simulink model "IEEE33BusTestSystemSimple"  (Simulink 10.3)
settings: Solver=FixedStepAuto  StartTime=0.0  StopTime=0.2  RelTol=1e-3
undefined symbols (not defined in the file): D1, Delta
libraries: spsThreePhaseVIMeasurementLib x43, spsThreePhaseSeriesRLCBranchLib x39, spsThreePhaseSeriesRLCLoadLib x34, simulink_extras x9, spsFrequencyPhasorLib x9, spsPowerPositiveSequenceLib x9, spsSequenceAnalyzerLib x9, spsThreePhaseParallelRLCLoadLib x3, spsSeriesRLCBranchLib x3, spsAC1AExcitationSystemLib x2, spsDieselMotorModel x2, spsSynchronousMachinepuStandardLib x2
(part 3 of 3)

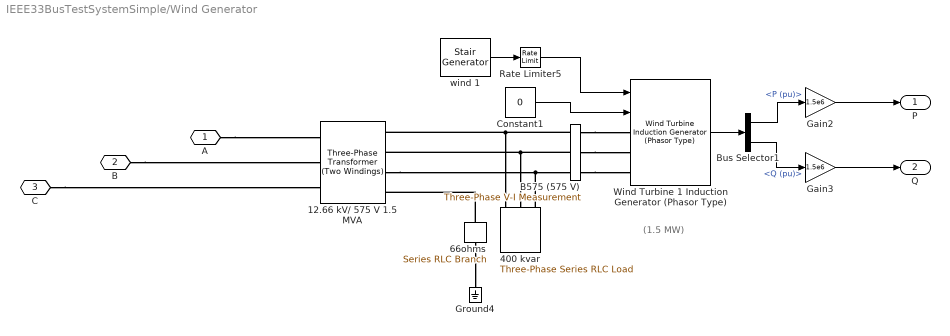
== system IEEE33BusTestSystemSimple/Wind Generator ==
  note: (1.5 MW)
  12.66 kV/ 575 V 1.5 MVA : spsThreePhaseTransformerTwoWindingsLib/Three-Phase Transformer (Two Windings)  Winding1Connection=Yg  Winding2Connection=Yn  CoreType=Three single-phase transformers  SetSaturation=off  Hysteresis=off  DataFile='hysteresis'  SetInitialFlux=off  Measurements=None  UNITS=pu  NominalPower="[1.5e6  50]"  Winding1=[12.66e3 , 0.025/30 , 0.025]  Winding2=[ 575, 0.025/30 , 0.025]  Rm=500  Lm=inf  L0=0.5  Saturation=[ 0,0 ; 0.0024,1.2 ; 1.0,1.52 ]  InitialFluxes=[ 0.8 , -0.8 , 0.7 ]  BreakLoop=off  DiscreteSolver=Trapezoidal iterative  DataType=off  TransfoNumber=0
  400 kvar : spsThreePhaseSeriesRLCLoadLib/Three-Phase Series RLC Load  LConnTagsString=A|B|C  Configuration=Delta  NominalVoltage=575  Vabc=[1e3 1e3 1e3]  Vabcp=[1e3 1e3 1e3]  NominalFrequency=50  UnbalancedPower=off  ActivePower=0  InductivePower=0  CapacitivePower=400e3  Pabc=[10e3 9e3 11e3]  QLabc=[100 90 110]  QCabc=[100 90 110]  Pabcp=[10e3 9e3 11e3]  QLabcp=[100 90 110]  QCabcp=[100 90 110]  Measurements=None  LoadType=constant Z
  "66ohms " : spsSeriesRLCBranchLib/Series RLC Branch  LConnTagsString=__new0  RConnTagsString=__new0  BranchType=R  Resistance=66  Inductance=1.0  SetiL0=off  InitialCurrent=0  Capacitance=1.0  Setx0=off  InitialVoltage=0  Measurements=None
  B575 (575 V) : spsThreePhaseVIMeasurementLib/Three-Phase V-I Measurement  VoltageMeasurement=phase-to-ground  SetLabelV=on  LabelV=Vabc_B575  Vpu=on  VpuLL=off  CurrentMeasurement=yes  SetLabelI=on  LabelI=Iabc_B575  Ipu=on  Pbase=1.5e6/0.9  Vbase=575  OutputType=Complex  PhasorSimulation=off  PSBequivalent=0
  Bus Selector1 : BusSelector  OutputSignals=P (pu),Q (pu)
  Constant1 : Constant  Value=0
  Gain2 : Gain  Gain=1.5e6
  Gain3 : Gain  Gain=1.5e6
  Ground4 : spsGroundLib/Ground  LConnTagsString=a
  Rate Limiter5 : RateLimiter
  Wind Turbine 1 Induction Generator (Phasor Type) : spsWindTurbineInductionGeneratorPhasorTypeLib/Wind Turbine Induction Generator (Phasor Type)  ExternalTm=off  nom=[1.5e6/0.9 575 50]  sta=[ 0.004843 0.1248]  rot=[ 0.004377 0.1791]  Lm=6.77  mec=[5.04 0.01 3]  init="[ -0.01,0   0,0,0   0,0,0 ]"  pitch_angle=0  Pmec=1.5e6  wind_base=9  speed_nom=1  P_wind_base=1  K_pitch_gain=[5 25]  pitch_max=45  pitch_rate=2
      settings: SourceProductBaseCode=PS
  wind 1 : spsStairGeneratorLib/Stair Generator  t=[ 0 2]  e=[8 12]  Ts=0
  A : PMIOPort  Side=Left
  B : PMIOPort  Port=2  Side=Left
  C : PMIOPort  Port=3  Side=Left
  P : Outport  VectorParamsAs1DForOutWhenUnconnected=off
  Q : Outport  Port=2  VectorParamsAs1DForOutWhenUnconnected=off
  wires:
  wind 1/1 -> Rate Limiter5/1
  Constant1/1 -> Wind Turbine 1 Induction Generator (Phasor Type)/2
  Rate Limiter5/1 -> Wind Turbine 1 Induction Generator (Phasor Type)/1
  Wind Turbine 1 Induction Generator (Phasor Type)/1 -> Bus Selector1/1
  Bus Selector1/1 -> Gain2/1  "<P (pu)>"
  Gain2/1 -> P/1
  Bus Selector1/2 -> Gain3/1  "<Q (pu)>"
  Gain3/1 -> Q/1
  connections:
  A/RConn1 -- 12.66 kV/ 575 V 1.5 MVA/LConn1
  12.66 kV/ 575 V 1.5 MVA/RConn3 -- 400 kvar/LConn3 -- B575 (575 V)/LConn3
  "66ohms "/RConn1 -- Ground4/LConn1
  B575 (575 V)/LConn2 -- 400 kvar/LConn2 -- 12.66 kV/ 575 V 1.5 MVA/RConn2
  B575 (575 V)/LConn1 -- 400 kvar/LConn1 -- 12.66 kV/ 575 V 1.5 MVA/RConn1
  "66ohms "/LConn1 -- 12.66 kV/ 575 V 1.5 MVA/RConn4
  B575 (575 V)/RConn3 -- Wind Turbine 1 Induction Generator (Phasor Type)/LConn3
  B575 (575 V)/RConn1 -- Wind Turbine 1 Induction Generator (Phasor Type)/LConn1
  B575 (575 V)/RConn2 -- Wind Turbine 1 Induction Generator (Phasor Type)/LConn2
  C/RConn1 -- 12.66 kV/ 575 V 1.5 MVA/LConn3
  B/RConn1 -- 12.66 kV/ 575 V 1.5 MVA/LConn2

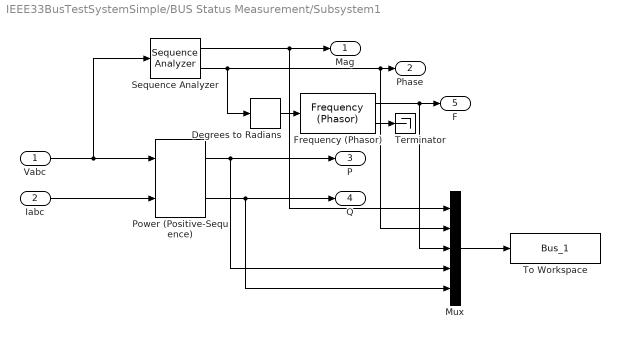
== system IEEE33BusTestSystemSimple/BUS Status Measurement/Subsystem1 ==
  Vabc : Inport
  Iabc : Inport  Port=2
  Degrees to Radians : simulink_extras/Transformations/Degrees to Radians
  Frequency (Phasor) : spsFrequencyPhasorLib/Frequency (Phasor)  Fn=50  T=0.1
      settings: SourceProductBaseCode=PS
  Mux : Mux  Inputs=5
  Power (Positive-Sequence) : spsPowerPositiveSequenceLib/Power (Positive-Sequence)  Freq=50  Vinit=[0, 0]  Iinit=[0, 0]  Ts=0
      settings: SourceProductBaseCode=PS
  Sequence Analyzer : spsSequenceAnalyzerLib/Sequence Analyzer  Freq=50  n=1  seq=Positive  InInit=[0, 0]  Ts=0
      settings: SourceProductBaseCode=PS
  Terminator : Terminator
  To Workspace : ToWorkspace  VariableName=Bus_1  SaveFormat=Timeseries  SampleTime=-1
  Mag : Outport
  Phase : Outport  Port=2
  P : Outport  Port=3
  Q : Outport  Port=4
  F : Outport  Port=5
  wires:
  Vabc/1 -> Sequence Analyzer/1, Power (Positive-Sequence)/1
  Power (Positive-Sequence)/2 -> Q/1, Mux/5
  Iabc/1 -> Power (Positive-Sequence)/2
  Power (Positive-Sequence)/1 -> P/1, Mux/4
  Sequence Analyzer/2 -> Mux/2, Phase/1, Degrees to Radians/1
  Sequence Analyzer/1 -> Mux/1, Mag/1
  Degrees to Radians/1 -> Frequency (Phasor)/1
  Frequency (Phasor)/1 -> Mux/3, F/1
  Frequency (Phasor)/2 -> Terminator/1
  Mux/1 -> To Workspace/1

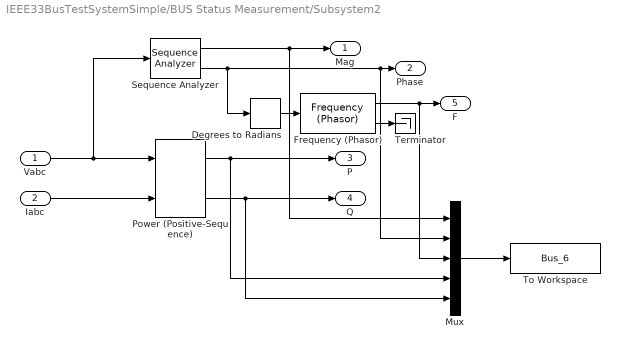
== system IEEE33BusTestSystemSimple/BUS Status Measurement/Subsystem2 ==
  Vabc : Inport
  Iabc : Inport  Port=2
  Degrees to Radians : simulink_extras/Transformations/Degrees to Radians
  Frequency (Phasor) : spsFrequencyPhasorLib/Frequency (Phasor)  Fn=50  T=0.1
      settings: SourceProductBaseCode=PS
  Mux : Mux  Inputs=5
  Power (Positive-Sequence) : spsPowerPositiveSequenceLib/Power (Positive-Sequence)  Freq=50  Vinit=[0, 0]  Iinit=[0, 0]  Ts=0
      settings: SourceProductBaseCode=PS
  Sequence Analyzer : spsSequenceAnalyzerLib/Sequence Analyzer  Freq=50  n=1  seq=Positive  InInit=[0, 0]  Ts=0
      settings: SourceProductBaseCode=PS
  Terminator : Terminator
  To Workspace : ToWorkspace  VariableName=Bus_6  SaveFormat=Timeseries  SampleTime=-1
  Mag : Outport
  Phase : Outport  Port=2
  P : Outport  Port=3
  Q : Outport  Port=4
  F : Outport  Port=5
  wires:
  Vabc/1 -> Sequence Analyzer/1, Power (Positive-Sequence)/1
  Iabc/1 -> Power (Positive-Sequence)/2
  Degrees to Radians/1 -> Frequency (Phasor)/1
  Frequency (Phasor)/2 -> Terminator/1
  Sequence Analyzer/1 -> Mux/1, Mag/1
  Mux/1 -> To Workspace/1
  Power (Positive-Sequence)/2 -> Mux/5, Q/1
  Frequency (Phasor)/1 -> Mux/3, F/1
  Sequence Analyzer/2 -> Mux/2, Phase/1, Degrees to Radians/1
  Power (Positive-Sequence)/1 -> Mux/4, P/1

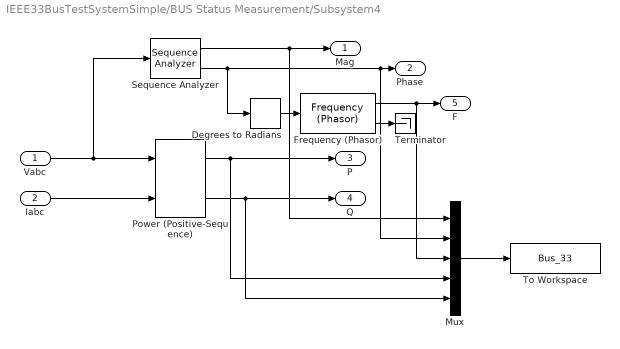
== system IEEE33BusTestSystemSimple/BUS Status Measurement/Subsystem4 ==
  Vabc : Inport
  Iabc : Inport  Port=2
  Degrees to Radians : simulink_extras/Transformations/Degrees to Radians
  Frequency (Phasor) : spsFrequencyPhasorLib/Frequency (Phasor)  Fn=50  T=0.1
      settings: SourceProductBaseCode=PS
  Mux : Mux  Inputs=5
  Power (Positive-Sequence) : spsPowerPositiveSequenceLib/Power (Positive-Sequence)  Freq=50  Vinit=[0, 0]  Iinit=[0, 0]  Ts=0
      settings: SourceProductBaseCode=PS
  Sequence Analyzer : spsSequenceAnalyzerLib/Sequence Analyzer  Freq=50  n=1  seq=Positive  InInit=[0, 0]  Ts=0
      settings: SourceProductBaseCode=PS
  Terminator : Terminator
  To Workspace : ToWorkspace  VariableName=Bus_33  SaveFormat=Timeseries  SampleTime=-1
  Mag : Outport
  Phase : Outport  Port=2
  P : Outport  Port=3
  Q : Outport  Port=4
  F : Outport  Port=5
  wires:
  Vabc/1 -> Sequence Analyzer/1, Power (Positive-Sequence)/1
  Iabc/1 -> Power (Positive-Sequence)/2
  Degrees to Radians/1 -> Frequency (Phasor)/1
  Frequency (Phasor)/2 -> Terminator/1
  Sequence Analyzer/1 -> Mux/1, Mag/1
  Mux/1 -> To Workspace/1
  Power (Positive-Sequence)/2 -> Mux/5, Q/1
  Frequency (Phasor)/1 -> Mux/3, F/1
  Sequence Analyzer/2 -> Mux/2, Phase/1, Degrees to Radians/1
  Power (Positive-Sequence)/1 -> Mux/4, P/1

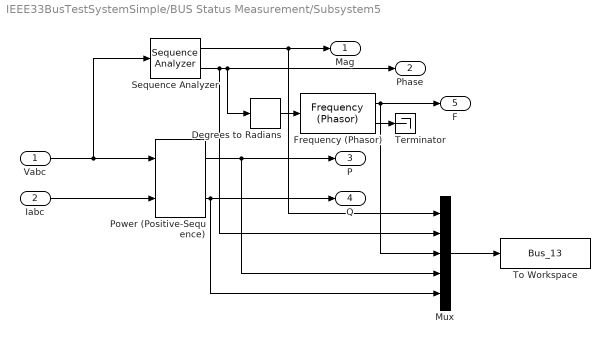
== system IEEE33BusTestSystemSimple/BUS Status Measurement/Subsystem5 ==
  Vabc : Inport
  Iabc : Inport  Port=2
  Degrees to Radians : simulink_extras/Transformations/Degrees to Radians
  Frequency (Phasor) : spsFrequencyPhasorLib/Frequency (Phasor)  Fn=50  T=0.1
      settings: SourceProductBaseCode=PS
  Mux : Mux  Inputs=5
  Power (Positive-Sequence) : spsPowerPositiveSequenceLib/Power (Positive-Sequence)  Freq=50  Vinit=[0, 0]  Iinit=[0, 0]  Ts=0
      settings: SourceProductBaseCode=PS
  Sequence Analyzer : spsSequenceAnalyzerLib/Sequence Analyzer  Freq=50  n=1  seq=Positive  InInit=[0, 0]  Ts=0
      settings: SourceProductBaseCode=PS
  Terminator : Terminator
  To Workspace : ToWorkspace  VariableName=Bus_13  SaveFormat=Timeseries  SampleTime=-1
  Mag : Outport
  Phase : Outport  Port=2
  P : Outport  Port=3
  Q : Outport  Port=4
  F : Outport  Port=5
  wires:
  Vabc/1 -> Sequence Analyzer/1, Power (Positive-Sequence)/1
  Iabc/1 -> Power (Positive-Sequence)/2
  Degrees to Radians/1 -> Frequency (Phasor)/1
  Frequency (Phasor)/2 -> Terminator/1
  Sequence Analyzer/1 -> Mux/1, Mag/1
  Mux/1 -> To Workspace/1
  Power (Positive-Sequence)/2 -> Mux/5, Q/1
  Frequency (Phasor)/1 -> Mux/3, F/1
  Sequence Analyzer/2 -> Mux/2, Phase/1, Degrees to Radians/1
  Power (Positive-Sequence)/1 -> Mux/4, P/1

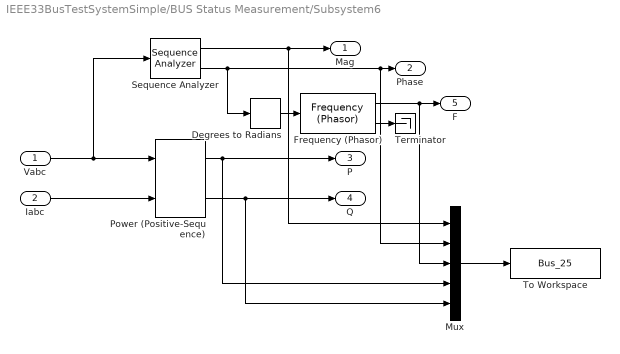
== system IEEE33BusTestSystemSimple/BUS Status Measurement/Subsystem6 ==
  Vabc : Inport
  Iabc : Inport  Port=2
  Degrees to Radians : simulink_extras/Transformations/Degrees to Radians
  Frequency (Phasor) : spsFrequencyPhasorLib/Frequency (Phasor)  Fn=50  T=0.1
      settings: SourceProductBaseCode=PS
  Mux : Mux  Inputs=5
  Power (Positive-Sequence) : spsPowerPositiveSequenceLib/Power (Positive-Sequence)  Freq=50  Vinit=[0, 0]  Iinit=[0, 0]  Ts=0
      settings: SourceProductBaseCode=PS
  Sequence Analyzer : spsSequenceAnalyzerLib/Sequence Analyzer  Freq=50  n=1  seq=Positive  InInit=[0, 0]  Ts=0
      settings: SourceProductBaseCode=PS
  Terminator : Terminator
  To Workspace : ToWorkspace  VariableName=Bus_25  SaveFormat=Timeseries  SampleTime=-1
  Mag : Outport
  Phase : Outport  Port=2
  P : Outport  Port=3
  Q : Outport  Port=4
  F : Outport  Port=5
  wires:
  Vabc/1 -> Sequence Analyzer/1, Power (Positive-Sequence)/1
  Iabc/1 -> Power (Positive-Sequence)/2
  Degrees to Radians/1 -> Frequency (Phasor)/1
  Frequency (Phasor)/2 -> Terminator/1
  Sequence Analyzer/1 -> Mux/1, Mag/1
  Mux/1 -> To Workspace/1
  Power (Positive-Sequence)/2 -> Mux/5, Q/1
  Frequency (Phasor)/1 -> Mux/3, F/1
  Sequence Analyzer/2 -> Mux/2, Phase/1, Degrees to Radians/1
  Power (Positive-Sequence)/1 -> Mux/4, P/1

== system IEEE33BusTestSystemSimple/Bus_10/VI Recorder13 ==
  Vrec : Inport
  Irec : Inport  Port=2
  tag scope: I9to10=global, V9to10=global
  wires:
  Vrec/1 -> [V9to10]
  Irec/1 -> [I9to10]

== system IEEE33BusTestSystemSimple/Bus_11/VI Recorder14 ==
  Vrec : Inport
  Irec : Inport  Port=2
  tag scope: I10to11=global, V10to11=global
  wires:
  Vrec/1 -> [V10to11]
  Irec/1 -> [I10to11]

== system IEEE33BusTestSystemSimple/Bus_12/VI Recorder15 ==
  Vrec : Inport
  Irec : Inport  Port=2
  tag scope: I11to12=global, V11to12=global
  wires:
  Vrec/1 -> [V11to12]
  Irec/1 -> [I11to12]

== system IEEE33BusTestSystemSimple/Bus_13/VI Recorder16 ==
  Vrec : Inport
  Irec : Inport  Port=2
  tag scope: I12to13=global, V12to13=global
  wires:
  Vrec/1 -> [V12to13]
  Irec/1 -> [I12to13]

== system IEEE33BusTestSystemSimple/Bus_14/VI Recorder17 ==
  Vrec : Inport
  Irec : Inport  Port=2
  tag scope: I13to14=global, V13to14=global
  wires:
  Vrec/1 -> [V13to14]
  Irec/1 -> [I13to14]

== system IEEE33BusTestSystemSimple/Bus_15/VI Recorder18 ==
  Vrec : Inport
  Irec : Inport  Port=2
  tag scope: I14to15=global, V14to15=global
  wires:
  Vrec/1 -> [V14to15]
  Irec/1 -> [I14to15]

== system IEEE33BusTestSystemSimple/Bus_16/VI Recorder19 ==
  Vrec : Inport
  Irec : Inport  Port=2
  tag scope: I15to16=global, V15to16=global
  wires:
  Vrec/1 -> [V15to16]
  Irec/1 -> [I15to16]

== system IEEE33BusTestSystemSimple/Bus_17/VI Recorder20 ==
  Vrec : Inport
  Irec : Inport  Port=2
  tag scope: I16to17=global, V16to17=global
  wires:
  Vrec/1 -> [V16to17]
  Irec/1 -> [I16to17]

== system IEEE33BusTestSystemSimple/Bus_18/VI Recorder21 ==
  Vrec : Inport
  Irec : Inport  Port=2
  tag scope: I17to18=global, V17to18=global
  wires:
  Vrec/1 -> [V17to18]
  Irec/1 -> [I17to18]

== system IEEE33BusTestSystemSimple/Bus_19/VI Recorder ==
  Vrec : Inport
  Irec : Inport  Port=2
  tag scope: I2to19=global, V2to19=global
  wires:
  Vrec/1 -> [V2to19]
  Irec/1 -> [I2to19]

== system IEEE33BusTestSystemSimple/Bus_2/VI Recorder5 ==
  Vrec : Inport
  Irec : Inport  Port=2
  tag scope: I1to2=global, V1to2=global
  wires:
  Vrec/1 -> [V1to2]
  Irec/1 -> [I1to2]

== system IEEE33BusTestSystemSimple/Bus_20/VI Recorder1 ==
  Vrec : Inport
  Irec : Inport  Port=2
  tag scope: I19to20=global, V19to20=global
  wires:
  Vrec/1 -> [V19to20]
  Irec/1 -> [I19to20]

== system IEEE33BusTestSystemSimple/Bus_21/VI Recorder2 ==
  Vrec : Inport
  Irec : Inport  Port=2
  tag scope: I20to21=global, V20to21=global
  wires:
  Vrec/1 -> [V20to21]
  Irec/1 -> [I20to21]

== system IEEE33BusTestSystemSimple/Bus_22/VI Recorder3 ==
  Vrec : Inport
  Irec : Inport  Port=2
  tag scope: I21to22=global, V21to22=global
  wires:
  Vrec/1 -> [V21to22]
  Irec/1 -> [I21to22]

== system IEEE33BusTestSystemSimple/Bus_23/VI Recorder32 ==
  Vrec : Inport
  Irec : Inport  Port=2
  tag scope: I3to23=global, V3to23=global
  wires:
  Vrec/1 -> [V3to23]
  Irec/1 -> [I3to23]

== system IEEE33BusTestSystemSimple/Bus_24/VI Recorder31 ==
  Vrec : Inport
  Irec : Inport  Port=2
  tag scope: I23to24=global, V23to24=global
  wires:
  Vrec/1 -> [V23to24]
  Irec/1 -> [I23to24]

== system IEEE33BusTestSystemSimple/Bus_25/VI Recorder30 ==
  Vrec : Inport
  Irec : Inport  Port=2
  tag scope: I24to25=global, V24to25=global
  wires:
  Vrec/1 -> [V24to25]
  Irec/1 -> [I24to25]

== system IEEE33BusTestSystemSimple/Bus_26/VI Recorder22 ==
  Vrec : Inport
  Irec : Inport  Port=2
  tag scope: I6to26=global, V6to26=global
  wires:
  Vrec/1 -> [V6to26]
  Irec/1 -> [I6to26]

== system IEEE33BusTestSystemSimple/Bus_27/VI Recorder23 ==
  Vrec : Inport
  Irec : Inport  Port=2
  tag scope: I26to27=global, V26to27=global
  wires:
  Vrec/1 -> [V26to27]
  Irec/1 -> [I26to27]

== system IEEE33BusTestSystemSimple/Bus_28/VI Recorder24 ==
  Vrec : Inport
  Irec : Inport  Port=2
  tag scope: I27to28=global, V27to28=global
  wires:
  Vrec/1 -> [V27to28]
  Irec/1 -> [I27to28]

== system IEEE33BusTestSystemSimple/Bus_29/VI Recorder25 ==
  Vrec : Inport
  Irec : Inport  Port=2
  tag scope: I28to29=global, V28to29=global
  wires:
  Vrec/1 -> [V28to29]
  Irec/1 -> [I28to29]

== system IEEE33BusTestSystemSimple/Bus_3/VI Recorder6 ==
  Vrec : Inport
  Irec : Inport  Port=2
  tag scope: I2to3=global, V2to3=global
  wires:
  Vrec/1 -> [V2to3]
  Irec/1 -> [I2to3]

== system IEEE33BusTestSystemSimple/Bus_30/VI Recorder26 ==
  Vrec : Inport
  Irec : Inport  Port=2
  tag scope: I29to30=global, V29to30=global
  wires:
  Vrec/1 -> [V29to30]
  Irec/1 -> [I29to30]

== system IEEE33BusTestSystemSimple/Bus_31/VI Recorder27 ==
  Vrec : Inport
  Irec : Inport  Port=2
  tag scope: I30to31=global, V30to31=global
  wires:
  Vrec/1 -> [V30to31]
  Irec/1 -> [I30to31]

== system IEEE33BusTestSystemSimple/Bus_32/VI Recorder28 ==
  Vrec : Inport
  Irec : Inport  Port=2
  tag scope: I31to32=global, V31to32=global
  wires:
  Vrec/1 -> [V31to32]
  Irec/1 -> [I31to32]

== system IEEE33BusTestSystemSimple/Bus_33/VI Recorder29 ==
  Vrec : Inport
  Irec : Inport  Port=2
  tag scope: I32to33=global, V32to33=global
  wires:
  Vrec/1 -> [V32to33]
  Irec/1 -> [I32to33]

== system IEEE33BusTestSystemSimple/Bus_4/VI Recorder7 ==
  Vrec : Inport
  Irec : Inport  Port=2
  tag scope: I3to4=global, V3to4=global
  wires:
  Vrec/1 -> [V3to4]
  Irec/1 -> [I3to4]

== system IEEE33BusTestSystemSimple/Bus_5/VI Recorder8 ==
  Vrec : Inport
  Irec : Inport  Port=2
  tag scope: I4to5=global, V4to5=global
  wires:
  Vrec/1 -> [V4to5]
  Irec/1 -> [I4to5]

== system IEEE33BusTestSystemSimple/Bus_6/VI Recorder9 ==
  Vrec : Inport
  Irec : Inport  Port=2
  tag scope: I5to6=global, V5to6=global
  wires:
  Vrec/1 -> [V5to6]
  Irec/1 -> [I5to6]

== system IEEE33BusTestSystemSimple/Bus_7/VI Recorder10 ==
  Vrec : Inport
  Irec : Inport  Port=2
  tag scope: I6to7=global, V6to7=global
  wires:
  Vrec/1 -> [V6to7]
  Irec/1 -> [I6to7]

== system IEEE33BusTestSystemSimple/Bus_8/VI Recorder11 ==
  Vrec : Inport
  Irec : Inport  Port=2
  tag scope: I7to8=global, V7to8=global
  wires:
  Vrec/1 -> [V7to8]
  Irec/1 -> [I7to8]

== system IEEE33BusTestSystemSimple/Bus_9/VI Recorder12 ==
  Vrec : Inport
  Irec : Inport  Port=2
  tag scope: I8to9=global, V8to9=global
  wires:
  Vrec/1 -> [V8to9]
  Irec/1 -> [I8to9]

== system IEEE33BusTestSystemSimple/DG Systems Status/Subsystem1 ==
  Vabc : Inport
  Iabc : Inport  Port=2
  Degrees to Radians : simulink_extras/Transformations/Degrees to Radians
  Frequency (Phasor) : spsFrequencyPhasorLib/Frequency (Phasor)  Fn=50  T=0.1
      settings: SourceProductBaseCode=PS
  Power (Positive-Sequence) : spsPowerPositiveSequenceLib/Power (Positive-Sequence)  Freq=50  Vinit=[0, 0]  Iinit=[0, 0]  Ts=0
      settings: SourceProductBaseCode=PS
  Sequence Analyzer : spsSequenceAnalyzerLib/Sequence Analyzer  Freq=50  n=1  seq=Positive  InInit=[0, 0]  Ts=0
      settings: SourceProductBaseCode=PS
  Terminator : Terminator
  Mag : Outport
  Phase : Outport  Port=2
  P : Outport  Port=3
  Q : Outport  Port=4
  F : Outport  Port=5
  wires:
  Vabc/1 -> Sequence Analyzer/1, Power (Positive-Sequence)/1
  Power (Positive-Sequence)/2 -> Q/1
  Iabc/1 -> Power (Positive-Sequence)/2
  Power (Positive-Sequence)/1 -> P/1
  Sequence Analyzer/2 -> Phase/1, Degrees to Radians/1
  Sequence Analyzer/1 -> Mag/1
  Degrees to Radians/1 -> Frequency (Phasor)/1
  Frequency (Phasor)/1 -> F/1
  Frequency (Phasor)/2 -> Terminator/1

== system IEEE33BusTestSystemSimple/DG Systems Status/Subsystem2 ==
  Vabc : Inport
  Iabc : Inport  Port=2
  Degrees to Radians : simulink_extras/Transformations/Degrees to Radians
  Frequency (Phasor) : spsFrequencyPhasorLib/Frequency (Phasor)  Fn=50  T=0.1
      settings: SourceProductBaseCode=PS
  Power (Positive-Sequence) : spsPowerPositiveSequenceLib/Power (Positive-Sequence)  Freq=50  Vinit=[0, 0]  Iinit=[0, 0]  Ts=0
      settings: SourceProductBaseCode=PS
  Sequence Analyzer : spsSequenceAnalyzerLib/Sequence Analyzer  Freq=50  n=1  seq=Positive  InInit=[0, 0]  Ts=0
      settings: SourceProductBaseCode=PS
  Terminator : Terminator
  Mag : Outport
  Phase : Outport  Port=2
  P : Outport  Port=3
  Q : Outport  Port=4
  F : Outport  Port=5
  wires:
  Vabc/1 -> Sequence Analyzer/1, Power (Positive-Sequence)/1
  Power (Positive-Sequence)/2 -> Q/1
  Iabc/1 -> Power (Positive-Sequence)/2
  Power (Positive-Sequence)/1 -> P/1
  Sequence Analyzer/2 -> Phase/1, Degrees to Radians/1
  Sequence Analyzer/1 -> Mag/1
  Degrees to Radians/1 -> Frequency (Phasor)/1
  Frequency (Phasor)/1 -> F/1
  Frequency (Phasor)/2 -> Terminator/1

== system IEEE33BusTestSystemSimple/DG Systems Status/Subsystem3 ==
  Vabc : Inport
  Iabc : Inport  Port=2
  Degrees to Radians : simulink_extras/Transformations/Degrees to Radians
  Frequency (Phasor) : spsFrequencyPhasorLib/Frequency (Phasor)  Fn=50  T=0.1
      settings: SourceProductBaseCode=PS
  Power (Positive-Sequence) : spsPowerPositiveSequenceLib/Power (Positive-Sequence)  Freq=50  Vinit=[0, 0]  Iinit=[0, 0]  Ts=0
      settings: SourceProductBaseCode=PS
  Sequence Analyzer : spsSequenceAnalyzerLib/Sequence Analyzer  Freq=50  n=1  seq=Positive  InInit=[0, 0]  Ts=0
      settings: SourceProductBaseCode=PS
  Terminator : Terminator
  Mag : Outport
  Phase : Outport  Port=2
  P : Outport  Port=3
  Q : Outport  Port=4
  F : Outport  Port=5
  wires:
  Vabc/1 -> Sequence Analyzer/1, Power (Positive-Sequence)/1
  Power (Positive-Sequence)/2 -> Q/1
  Iabc/1 -> Power (Positive-Sequence)/2
  Power (Positive-Sequence)/1 -> P/1
  Sequence Analyzer/2 -> Phase/1, Degrees to Radians/1
  Sequence Analyzer/1 -> Mag/1
  Degrees to Radians/1 -> Frequency (Phasor)/1
  Frequency (Phasor)/1 -> F/1
  Frequency (Phasor)/2 -> Terminator/1

== system IEEE33BusTestSystemSimple/DG Systems Status/Subsystem4 ==
  Vabc : Inport
  Iabc : Inport  Port=2
  Degrees to Radians : simulink_extras/Transformations/Degrees to Radians
  Frequency (Phasor) : spsFrequencyPhasorLib/Frequency (Phasor)  Fn=50  T=0.1
      settings: SourceProductBaseCode=PS
  Power (Positive-Sequence) : spsPowerPositiveSequenceLib/Power (Positive-Sequence)  Freq=50  Vinit=[0, 0]  Iinit=[0, 0]  Ts=0
      settings: SourceProductBaseCode=PS
  Sequence Analyzer : spsSequenceAnalyzerLib/Sequence Analyzer  Freq=50  n=1  seq=Positive  InInit=[0, 0]  Ts=0
      settings: SourceProductBaseCode=PS
  Terminator : Terminator
  Mag : Outport
  Phase : Outport  Port=2
  P : Outport  Port=3
  Q : Outport  Port=4
  F : Outport  Port=5
  wires:
  Vabc/1 -> Sequence Analyzer/1, Power (Positive-Sequence)/1
  Power (Positive-Sequence)/2 -> Q/1
  Iabc/1 -> Power (Positive-Sequence)/2
  Power (Positive-Sequence)/1 -> P/1
  Sequence Analyzer/2 -> Phase/1, Degrees to Radians/1
  Sequence Analyzer/1 -> Mag/1
  Degrees to Radians/1 -> Frequency (Phasor)/1
  Frequency (Phasor)/1 -> F/1
  Frequency (Phasor)/2 -> Terminator/1

== system IEEE33BusTestSystemSimple/Diesel Generator 1/Generator Measures ==
  m : Inport
  Bus Selector : BusSelector  OutputSignals="dq0 components.Stator voltage  vq (pu),dq0 components.Stator voltage  vd (pu)"  OutputAsBus=on
  Bus Selector1 : BusSelector  OutputSignals="Mechanical.Rotor speed  wm  (pu),dq0 components.Field current  ifd (pu)"
  Fcn1 : Fcn  Expr=sqrt(u(1)^2 + u(2)^2)
  Ifd : Outport  VectorParamsAs1DForOutWhenUnconnected=off
  Vt : Outport  Port=2  VectorParamsAs1DForOutWhenUnconnected=off
  wm : Outport  Port=3  VectorParamsAs1DForOutWhenUnconnected=off
  wires:
  Bus Selector1/1 -> wm/1  "<Rotor speed  wm  (pu)>"
  m/1 -> Bus Selector1/1, Bus Selector/1
  Fcn1/1 -> Vt/1
  Bus Selector/1 -> Fcn1/1
  Bus Selector1/2 -> Ifd/1  "<Field current  ifd (pu)>"

== system IEEE33BusTestSystemSimple/Diesel Generator 1/Selected Measurements ==
  m : Inport
  Bus Creator : BusCreator  Inputs=7
  Bus Selector : BusSelector  OutputSignals="Mechanical.Electrical power  Pe (pu),Mechanical.Rotor speed  wm  (pu),Output active power   Peo (pu),Output reactive power  Qeo (pu)"
  to W : Gain  Gain=Pn
  to W1 : Gain  Gain=Pn
  to W2 : Gain  Gain=Pn
  sm : Outport  VectorParamsAs1DForOutWhenUnconnected=off
  wires:
  to W2/1 -> Bus Creator/7  "Reactive Power (W)"
  to W1/1 -> Bus Creator/6  "Active Power (W)"
  Bus Selector/2 -> Bus Creator/3  "<Rotor speed  wm  (pu)>"
  Bus Creator/1 -> sm/1
  to W/1 -> Bus Creator/1  "Electrical Power (W)"
  Bus Selector/3 -> Bus Creator/4, to W1/1  "<Output active power   Peo (pu)>"
  Bus Selector/1 -> to W/1, Bus Creator/2  "<Electrical power  Pe (pu)>"
  Bus Selector/4 -> Bus Creator/5, to W2/1  "<Output reactive power  Qeo (pu)>"
  m/1 -> Bus Selector/1

== system IEEE33BusTestSystemSimple/Diesel Generator 2/Generator Measures ==
  m : Inport
  Bus Selector : BusSelector  OutputSignals="dq0 components.Stator voltage  vq (pu),dq0 components.Stator voltage  vd (pu)"  OutputAsBus=on
  Bus Selector1 : BusSelector  OutputSignals="Mechanical.Rotor speed  wm  (pu),dq0 components.Field current  ifd (pu)"
  Fcn1 : Fcn  Expr=sqrt(u(1)^2 + u(2)^2)
  Ifd : Outport  VectorParamsAs1DForOutWhenUnconnected=off
  Vt : Outport  Port=2  VectorParamsAs1DForOutWhenUnconnected=off
  wm : Outport  Port=3  VectorParamsAs1DForOutWhenUnconnected=off
  wires:
  Bus Selector1/1 -> wm/1  "<Rotor speed  wm  (pu)>"
  m/1 -> Bus Selector1/1, Bus Selector/1
  Fcn1/1 -> Vt/1
  Bus Selector/1 -> Fcn1/1
  Bus Selector1/2 -> Ifd/1  "<Field current  ifd (pu)>"

== system IEEE33BusTestSystemSimple/Diesel Generator 2/Selected Measurements ==
  m : Inport
  Bus Creator : BusCreator  Inputs=7
  Bus Selector : BusSelector  OutputSignals="Mechanical.Electrical power  Pe (pu),Mechanical.Rotor speed  wm  (pu),Output active power   Peo (pu),Output reactive power  Qeo (pu)"
  to W : Gain  Gain=Pn
  to W1 : Gain  Gain=Pn
  to W2 : Gain  Gain=Pn
  sm : Outport  VectorParamsAs1DForOutWhenUnconnected=off
  wires:
  to W2/1 -> Bus Creator/7  "Reactive Power (W)"
  to W1/1 -> Bus Creator/6  "Active Power (W)"
  Bus Selector/2 -> Bus Creator/3  "<Rotor speed  wm  (pu)>"
  Bus Creator/1 -> sm/1
  to W/1 -> Bus Creator/1  "Electrical Power (W)"
  Bus Selector/3 -> Bus Creator/4, to W1/1  "<Output active power   Peo (pu)>"
  Bus Selector/1 -> to W/1, Bus Creator/2  "<Electrical power  Pe (pu)>"
  Bus Selector/4 -> Bus Creator/5, to W2/1  "<Output reactive power  Qeo (pu)>"
  m/1 -> Bus Selector/1

== system IEEE33BusTestSystemSimple/PV Array 2 /LC Filter ==
  C' : spsThreePhaseSeriesRLCBranchLib/Three-Phase Series RLC Branch  Commented=on  LConnTagsString=A|B|C  RConnTagsString=A|B|C  BranchType=C  Resistance=1e6  Inductance=500e-6/2  Capacitance=1e-3  Measurements=None
  L : spsThreePhaseSeriesRLCBranchLib/Three-Phase Series RLC Branch  LConnTagsString=A|B|C  RConnTagsString=A|B|C  BranchType=RL  Resistance=500e-6*377/50/2  Inductance=5*500e-6/2  Capacitance=inf  Measurements=None
  Three-Phase Series RLC Load : spsThreePhaseSeriesRLCLoadLib/Three-Phase Series RLC Load  LConnTagsString=A|B|C  Configuration=Y (grounded)  NominalVoltage=240  Vabc=[1e3 1e3 1e3]  Vabcp=[1e3 1e3 1e3]  NominalFrequency=50  UnbalancedPower=off  ActivePower=5*10e3/100  InductivePower=0  CapacitivePower=5*10e3  Pabc=[10e3 9e3 11e3]  QLabc=[100 90 110]  QCabc=[100 90 110]  Pabcp=[10e3 9e3 11e3]  QLabcp=[100 90 110]  QCabcp=[100 90 110]  Measurements=None  LoadType=constant Z
  A : PMIOPort  Side=Left
  a : PMIOPort  Port=2  Side=Right
  B : PMIOPort  Port=3  Side=Left
  b : PMIOPort  Port=4  Side=Right
  C : PMIOPort  Port=5  Side=Left
  c : PMIOPort  Port=6  Side=Right
  connections:
  c/RConn1 -- C'/LConn3 -- L/RConn3 -- Three-Phase Series RLC Load/LConn3
  C'/RConn1 -- C'/RConn3 -- C'/RConn2
  b/RConn1 -- L/RConn2 -- C'/LConn2 -- Three-Phase Series RLC Load/LConn2
  a/RConn1 -- C'/LConn1 -- L/RConn1 -- Three-Phase Series RLC Load/LConn1
  L/LConn3 -- C/RConn1
  L/LConn1 -- A/RConn1
  B/RConn1 -- L/LConn2

== system IEEE33BusTestSystemSimple/PV Array 2 /PWM ==
  Mux : Mux  Inputs=3
  PWM Generator (3-Level) : spsPWMGenerator3LevelLib/PWM Generator (3-Level)  ModulatorType=Three-phase bridge (12 pulses)  ModulatorMode=Unsynchronized  nF=27  Fc=27*50*3  ModulatingSignals=off  m=0.8  Freq=60  Phase=0  Ts=0
      settings: SourceProductBaseCode=PS
  Vref A : Sin  Frequency=2*pi*50  SampleTime=0
  Vref B : Sin  Frequency=2*pi*50  Phase=2*pi/3  SampleTime=0
  Vref C : Sin  Frequency=2*pi*50  Phase=4*pi/3  SampleTime=0
  pulse : Outport  VectorParamsAs1DForOutWhenUnconnected=off
  wires:
  Vref B/1 -> Mux/2
  Vref C/1 -> Mux/3
  PWM Generator (3-Level)/1 -> pulse/1
  Vref A/1 -> Mux/1
  Mux/1 -> PWM Generator (3-Level)/1
